simulink model "ES008A_PwrSply"  (R2013b)
settings: Solver=FixedStepDiscrete  SolverMode=SingleTasking  StartTime=0.0  StopTime=1  FixedStep=0.002  RelTol=1e-3
values from neighbouring files (symbols this model uses):
  DiagcReg0Err = DataDict.NTC    [ES008A_PwrSply_DataDict.m]
  DiagcReg1Err = DataDict.NTC    [ES008A_PwrSply_DataDict.m]
  PWRSPLYDIAGREG0READVAL_CNT_U16 = DataDict.Constant    [ES008A_PwrSply_DataDict.m]
  PWRSPLYDIAGREG1READVAL_CNT_U16 = DataDict.Constant    [ES008A_PwrSply_DataDict.m]
  PwrSplyNtc0x07BFailStep = DataDict.Calibration    [ES008A_PwrSply_DataDict.m]
  PwrSplyNtc0x07BPassStep = DataDict.Calibration    [ES008A_PwrSply_DataDict.m]
  PwrSplyNtc0x07CFailStep = DataDict.Calibration    [ES008A_PwrSply_DataDict.m]
  PwrSplyNtc0x07CPassStep = DataDict.Calibration    [ES008A_PwrSply_DataDict.m]
  PwrSplyNtc0x07DFailStep = DataDict.Calibration    [ES008A_PwrSply_DataDict.m]
  PwrSplyNtc0x07DPassStep = DataDict.Calibration    [ES008A_PwrSply_DataDict.m]
  PWRSPLYOUTPENAWRVAL_CNT_U16 = DataDict.Constant    [ES008A_PwrSply_DataDict.m]
  PWRSPLYVRFYRESREG0READVAL_CNT_U16 = DataDict.Constant    [ES008A_PwrSply_DataDict.m]
  PWRSPLYVRFYRESREG1READVAL_CNT_U16 = DataDict.Constant    [ES008A_PwrSply_DataDict.m]
  SerlErr = DataDict.NTC    [ES008A_PwrSply_DataDict.m]
  SpiConf_SpiChannel_PwrSplyCh1 = DataDict.Constant    [ES008A_PwrSply_DataDict.m]
  SpiConf_SpiChannel_PwrSplyCh2 = DataDict.Constant    [ES008A_PwrSply_DataDict.m]
  SpiConf_SpiChannel_PwrSplyCh3 = DataDict.Constant    [ES008A_PwrSply_DataDict.m]
  SpiConf_SpiChannel_PwrSplyCh4 = DataDict.Constant    [ES008A_PwrSply_DataDict.m]
  SpiConf_SpiChannel_PwrSplyCh5 = DataDict.Constant    [ES008A_PwrSply_DataDict.m]
  SpiConf_SpiSequence_PwrSplySeq1 = DataDict.Constant    [ES008A_PwrSply_DataDict.m]
  SpiConf_SpiSequence_PwrSplySeq2 = DataDict.Constant    [ES008A_PwrSply_DataDict.m]
  SpiConf_SpiSequence_PwrSplySeq3 = DataDict.Constant    [ES008A_PwrSply_DataDict.m]
  SpiConf_SpiSequence_PwrSplySeq4 = DataDict.Constant    [ES008A_PwrSply_DataDict.m]
  SpiConf_SpiSequence_PwrSplySeq5 = DataDict.Constant    [ES008A_PwrSply_DataDict.m]
  StrtUpSelfTestReg0Err = DataDict.NTC    [ES008A_PwrSply_DataDict.m]
  StrtUpSelfTestReg1Err = DataDict.NTC    [ES008A_PwrSply_DataDict.m]
undefined symbols (not defined in the file or in its folder): sigbuilder_block, SysSt1
libraries: simulink x11
(part 2 of 4)

== system ES008A_PwrSply/PwrSply/PwrSplyPer1/SysSt = Enable/PwrSplyReadWrOrderFlg1 = 1 (Read Buffer)/CH 2 // Diag Reg 0 Error - NTCNR_0X07C (V5P, V5A, V5B, V5CAN) ==
  note: Read Buffer: Temporal Monitor State
  note: Channel 2 --> for Diag Register 0
      | Channel 3 --> for Diag Register 1
  note: Diag Register 0
  Action Port : ActionPort  ActionType=then
  Chk Error : simulink/Logic and Bit Operations/Bitwise Operator  logicop=AND  UseBitMask=on  BitMask=bin2dec('11111111')  BitMaskRealWorld=Stored Integer
  Constant2 : Constant  Value=SpiConf_SpiChannel_PwrSplyCh2
  CopyRight1 : Subsystem  Description=|  mask(Copyright Information){none=on}
      | Copyright info block.                                               
      |                                                                     
      | Place copyright information at the top of every subsystem in design.
      mask prompts: none "No parameters"
      mask help: Place copyright information at the top of every subsystem in design.
      mask Display:
      | NxtrConf = 'Nexteer Confidential';
      | 
      | sys = bdroot; %handle for the current model ("system")
      | first = get_param(sys,'Created');
      | first = first(end-3:end);  %year is last four digits
      | 
      | last = get_param(sys,'LastModifiedDate');
      | if isempty(last)
      |     last = datestr(now,'yyyy');
      | else
      |     last = last(end-3:end);
      | end
      | 
      | if strcmp(first,last)
      |     fprintf('%s -- Copyright %s Nexteer',NxtrConf,first)
      | else
      |     fprintf('%s -- %s%s- %s Nexteer',NxtrConf,char(169),first,last)
      | end
  Debounce Step : Constant  Value=PwrSplyNtc0x07CFailStep  OutDataTypeStr=uint16
  NtcNr : Constant  Value=DiagcReg0Err
  NtcSts : Constant  Value=3  OutDataTypeStr=uint8
  SetNtcSts : Subsystem  RequirementInfo={'linktype_rmi_doors' '0000cf50 (/ESG Group/FDD Module Requirements/EA4 Specific/ES008A - PwrSply)' '#ES008A_90' 'true' 'REQ: ES008A_90' '' ; 'linktype_rmi_doors' '0000cf50 (/ESG Group/FDD Module Requirements/EA4 Specific/ES008A_PwrSply)' '#ES008A_111' 'true' 'REQ: ES008A_111' '' } %GIDa_0e611bfb_5a91_4369_9638_8556bad60356
  Spi_ReadIB : Subsystem  RequirementInfo={'linktype_rmi_doors' '0000cf50 (/ESG Group/FDD Module Requirements/EA4 Specific/ES008A_PwrSply)' '#ES008A_110' 'true' 'REQ: ES008A_110' '' } %GIDa_1744bced_b149_4c04_97ae_ac37b4232d20
  wires:
  NtcSts/1 -> SetNtcSts/3(NtcSts)
  Debounce Step/1 -> SetNtcSts/4(DebStep)
  NtcNr/1 -> SetNtcSts/1(NtcNr)
  Constant2/1 -> Spi_ReadIB/1(Channel)
  Spi_ReadIB/1(Rx) -> Chk Error/1
  Chk Error/1 -> SetNtcSts/2(NtcStInfo)

== system ES008A_PwrSply/PwrSply/PwrSplyPer1/SysSt = Enable/PwrSplyReadWrOrderFlg1 = 1 (Read Buffer)/CH 3 // Diag Reg 1 Error - NTCNR_0X07B (VREG, BUCK, V3V3) ==
  note: Channel 2 --> for Diag Register 0
      | Channel 3 --> for Diag Register 1
  note: Read Buffer: Temporal Monitor State
  note: Diag Register 1
  Action Port : ActionPort  ActionType=then
  Chk Error : simulink/Logic and Bit Operations/Bitwise Operator  logicop=AND  UseBitMask=on  BitMask=bin2dec('00111111')  BitMaskRealWorld=Stored Integer
  Constant2 : Constant  Value=SpiConf_SpiChannel_PwrSplyCh3
  CopyRight1 : Subsystem  Description=|  mask(Copyright Information){none=on}
      | Copyright info block.                                               
      |                                                                     
      | Place copyright information at the top of every subsystem in design.
      mask prompts: none "No parameters"
      mask help: Place copyright information at the top of every subsystem in design.
      mask Display:
      | NxtrConf = 'Nexteer Confidential';
      | 
      | sys = bdroot; %handle for the current model ("system")
      | first = get_param(sys,'Created');
      | first = first(end-3:end);  %year is last four digits
      | 
      | last = get_param(sys,'LastModifiedDate');
      | if isempty(last)
      |     last = datestr(now,'yyyy');
      | else
      |     last = last(end-3:end);
      | end
      | 
      | if strcmp(first,last)
      |     fprintf('%s -- Copyright %s Nexteer',NxtrConf,first)
      | else
      |     fprintf('%s -- %s%s- %s Nexteer',NxtrConf,char(169),first,last)
      | end
  Debounce Step : Constant  Value=PwrSplyNtc0x07BFailStep  OutDataTypeStr=uint16
  NtcNr : Constant  Value=DiagcReg1Err
  NtcSts : Constant  Value=3  OutDataTypeStr=uint8
  SetNtcSts : Subsystem  RequirementInfo={'linktype_rmi_doors' '0000cf50 (/ESG Group/FDD Module Requirements/EA4 Specific/ES008A - PwrSply)' '#ES008A_22' 'true' 'REQ: ES008A_22' '' ; 'linktype_rmi_doors' '0000cf50 (/ESG Group/FDD Module Requirements/EA4 Specific/ES008A_PwrSply)' '#ES008A_111' 'true' 'REQ: ES008A_111' '' } %GIDa_0332d9c1_390b_4a00_b6d5_767a4bc1c83a
  Spi_ReadIB : Subsystem  RequirementInfo={'linktype_rmi_doors' '0000cf50 (/ESG Group/FDD Module Requirements/EA4 Specific/ES008A_PwrSply)' '#ES008A_110' 'true' 'REQ: ES008A_110' '' } %GIDa_30f8a1e3_071e_4be7_af63_a65be91c4651
  wires:
  Chk Error/1 -> SetNtcSts/2(NtcStInfo)
  Spi_ReadIB/1(Rx) -> Chk Error/1
  Constant2/1 -> Spi_ReadIB/1(Channel)
  NtcNr/1 -> SetNtcSts/1(NtcNr)
  Debounce Step/1 -> SetNtcSts/4(DebStep)
  NtcSts/1 -> SetNtcSts/3(NtcSts)

== system ES008A_PwrSply/PwrSply/PwrSplyPer1/SysSt = Enable/PwrSplyReadWrOrderFlg1 = 1 (Read Buffer)/CopyRight1 ==

== system ES008A_PwrSply/PwrSply/PwrSplyPer1/SysSt = Enable/PwrSplyReadWrOrderFlg1 = 1 (Read Buffer)/No  Error - Diag Reg 0 ==
  Action Port : ActionPort  ActionType=else
  CopyRight1 : Subsystem  Description=|  mask(Copyright Information){none=on}
      | Copyright info block.                                               
      |                                                                     
      | Place copyright information at the top of every subsystem in design.
      mask prompts: none "No parameters"
      mask help: Place copyright information at the top of every subsystem in design.
      mask Display:
      | NxtrConf = 'Nexteer Confidential';
      | 
      | sys = bdroot; %handle for the current model ("system")
      | first = get_param(sys,'Created');
      | first = first(end-3:end);  %year is last four digits
      | 
      | last = get_param(sys,'LastModifiedDate');
      | if isempty(last)
      |     last = datestr(now,'yyyy');
      | else
      |     last = last(end-3:end);
      | end
      | 
      | if strcmp(first,last)
      |     fprintf('%s -- Copyright %s Nexteer',NxtrConf,first)
      | else
      |     fprintf('%s -- %s%s- %s Nexteer',NxtrConf,char(169),first,last)
      | end
  Debounce Step : Constant  Value=PwrSplyNtc0x07CPassStep  OutDataTypeStr=uint16
  NtcNr : Constant  Value=DiagcReg0Err
  NtcSts : Constant  Value=2  OutDataTypeStr=uint8
  NtcStsInfo : Constant  Value=0  OutDataTypeStr=uint8
  SetNtcSts : Subsystem
  wires:
  NtcSts/1 -> SetNtcSts/3(NtcSts)
  Debounce Step/1 -> SetNtcSts/4(DebStep)
  NtcNr/1 -> SetNtcSts/1(NtcNr)
  NtcStsInfo/1 -> SetNtcSts/2(NtcStInfo)

== system ES008A_PwrSply/PwrSply/PwrSplyPer1/SysSt = Enable/PwrSplyReadWrOrderFlg1 = 1 (Read Buffer)/No  Error - Diag Reg 1 ==
  Action Port : ActionPort  ActionType=else
  CopyRight1 : Subsystem  Description=|  mask(Copyright Information){none=on}
      | Copyright info block.                                               
      |                                                                     
      | Place copyright information at the top of every subsystem in design.
      mask prompts: none "No parameters"
      mask help: Place copyright information at the top of every subsystem in design.
      mask Display:
      | NxtrConf = 'Nexteer Confidential';
      | 
      | sys = bdroot; %handle for the current model ("system")
      | first = get_param(sys,'Created');
      | first = first(end-3:end);  %year is last four digits
      | 
      | last = get_param(sys,'LastModifiedDate');
      | if isempty(last)
      |     last = datestr(now,'yyyy');
      | else
      |     last = last(end-3:end);
      | end
      | 
      | if strcmp(first,last)
      |     fprintf('%s -- Copyright %s Nexteer',NxtrConf,first)
      | else
      |     fprintf('%s -- %s%s- %s Nexteer',NxtrConf,char(169),first,last)
      | end
  Debounce Step : Constant  Value=PwrSplyNtc0x07BPassStep  OutDataTypeStr=uint16
  NtcNr : Constant  Value=DiagcReg1Err
  NtcSts : Constant  Value=2  OutDataTypeStr=uint8
  NtcStsInfo : Constant  Value=0  OutDataTypeStr=uint8
  SetNtcSts : Subsystem
  wires:
  NtcStsInfo/1 -> SetNtcSts/2(NtcStInfo)
  NtcNr/1 -> SetNtcSts/1(NtcNr)
  Debounce Step/1 -> SetNtcSts/4(DebStep)
  NtcSts/1 -> SetNtcSts/3(NtcSts)

== system ES008A_PwrSply/PwrSply/PwrSplyPer1/SysSt = Enable/PwrSplyReadWrOrderFlg1 = 1 (Read Buffer)/No Serial Error ==
  Action Port : ActionPort  ActionType=else
  CopyRight1 : Subsystem  Description=|  mask(Copyright Information){none=on}
      | Copyright info block.                                               
      |                                                                     
      | Place copyright information at the top of every subsystem in design.
      mask prompts: none "No parameters"
      mask help: Place copyright information at the top of every subsystem in design.
      mask Display:
      | NxtrConf = 'Nexteer Confidential';
      | 
      | sys = bdroot; %handle for the current model ("system")
      | first = get_param(sys,'Created');
      | first = first(end-3:end);  %year is last four digits
      | 
      | last = get_param(sys,'LastModifiedDate');
      | if isempty(last)
      |     last = datestr(now,'yyyy');
      | else
      |     last = last(end-3:end);
      | end
      | 
      | if strcmp(first,last)
      |     fprintf('%s -- Copyright %s Nexteer',NxtrConf,first)
      | else
      |     fprintf('%s -- %s%s- %s Nexteer',NxtrConf,char(169),first,last)
      | end
  Debounce Step : Constant  Value=PwrSplyNtc0x07DPassStep  OutDataTypeStr=uint16
  NtcNr : Constant  Value=SerlErr
  NtcSts : Constant  Value=2  OutDataTypeStr=uint8
  NtcStsInfo : Constant  Value=0  OutDataTypeStr=uint8
  SetNtcSts : Subsystem
  wires:
  NtcSts/1 -> SetNtcSts/3(NtcSts)
  Debounce Step/1 -> SetNtcSts/4(DebStep)
  NtcNr/1 -> SetNtcSts/1(NtcNr)
  NtcStsInfo/1 -> SetNtcSts/2(NtcStInfo)

== system ES008A_PwrSply/PwrSply/PwrSplyPer1/SysSt = Enable/PwrSplyReadWrOrderFlg1 = 1 (Read Buffer)/Serial Error - NTCNR_0X07D ==
  Action Port : ActionPort  ActionType=then
  CopyRight1 : Subsystem  Description=|  mask(Copyright Information){none=on}
      | Copyright info block.                                               
      |                                                                     
      | Place copyright information at the top of every subsystem in design.
      mask prompts: none "No parameters"
      mask help: Place copyright information at the top of every subsystem in design.
      mask Display:
      | NxtrConf = 'Nexteer Confidential';
      | 
      | sys = bdroot; %handle for the current model ("system")
      | first = get_param(sys,'Created');
      | first = first(end-3:end);  %year is last four digits
      | 
      | last = get_param(sys,'LastModifiedDate');
      | if isempty(last)
      |     last = datestr(now,'yyyy');
      | else
      |     last = last(end-3:end);
      | end
      | 
      | if strcmp(first,last)
      |     fprintf('%s -- Copyright %s Nexteer',NxtrConf,first)
      | else
      |     fprintf('%s -- %s%s- %s Nexteer',NxtrConf,char(169),first,last)
      | end
  Debounce Step : Constant  Value=PwrSplyNtc0x07DFailStep  OutDataTypeStr=uint16
  NtcNr : Constant  Value=SerlErr
  NtcSts : Constant  Value=3  OutDataTypeStr=uint8
  NtcSts1 : Constant  OutDataTypeStr=uint8
  SetNtcSts : Subsystem  RequirementInfo={'linktype_rmi_doors' '0000cf50 (/ESG Group/FDD Module Requirements/EA4 Specific/ES008A - PwrSply)' '#ES008A_96' 'true' 'REQ: ES008A_96' '' } %GIDa_f352822b_41ef_4404_b4d0_7ec6dffd63c0
  wires:
  NtcSts/1 -> SetNtcSts/3(NtcSts)
  Debounce Step/1 -> SetNtcSts/4(DebStep)
  NtcNr/1 -> SetNtcSts/1(NtcNr)
  NtcSts1/1 -> SetNtcSts/2(NtcStInfo)

== system ES008A_PwrSply/PwrSply/PwrSplyPer1/SysSt = Enable/PwrSplyReadWrOrderFlg1 = 1 (Read Buffer)/Spi_ReadIB ==
  note: 001011111111110
  note: Read Buffer - Simulation Purpose Only
  Channel : Inport
  Constant3 : Constant  Value=44  OutDataTypeStr=uint16
  CopyRight1 : Subsystem  Description=|  mask(Copyright Information){none=on}
      | Copyright info block.                                               
      |                                                                     
      | Place copyright information at the top of every subsystem in design.
      mask prompts: none "No parameters"
      mask help: Place copyright information at the top of every subsystem in design.
      mask Display:
      | NxtrConf = 'Nexteer Confidential';
      | 
      | sys = bdroot; %handle for the current model ("system")
      | first = get_param(sys,'Created');
      | first = first(end-3:end);  %year is last four digits
      | 
      | last = get_param(sys,'LastModifiedDate');
      | if isempty(last)
      |     last = datestr(now,'yyyy');
      | else
      |     last = last(end-3:end);
      | end
      | 
      | if strcmp(first,last)
      |     fprintf('%s -- Copyright %s Nexteer',NxtrConf,first)
      | else
      |     fprintf('%s -- %s%s- %s Nexteer',NxtrConf,char(169),first,last)
      | end
  Terminator : Terminator
  Rx : Outport
  wires:
  Constant3/1 -> Rx/1
  Channel/1 -> Terminator/1

== system ES008A_PwrSply/PwrSply/PwrSplyPer1/SysSt = Warm Init OR Enable/PwrSplyReadWrOrderFlg2 = 0 (Write Cmd to get Diag Status) /CopyRight1 ==

== system ES008A_PwrSply/PwrSply/PwrSplyPer1/SysSt = Warm Init OR Enable/PwrSplyReadWrOrderFlg2 = 0 (Write Cmd to get Diag Status) /Read Message 1 ==
  note: Read Cmd: Diag Reg 0: 01010 0 0 00000000 P
  note: Channel 4 --> for Verify_Result_0 Register
      | Channel 5 --> for Verify_Result_1 Register
  note: 10240
  Call_Spi_AsyncTransmit : Subsystem
  Constant2 : Constant  Value=SpiConf_SpiSequence_PwrSplySeq4
  Constant3 : Constant  Value=SpiConf_SpiChannel_PwrSplyCh4
  Constant5 : Constant  Value=PWRSPLYVRFYRESREG0READVAL_CNT_U16
  CopyRight1 : Subsystem  Description=|  mask(Copyright Information){none=on}
      | Copyright info block.                                               
      |                                                                     
      | Place copyright information at the top of every subsystem in design.
      mask prompts: none "No parameters"
      mask help: Place copyright information at the top of every subsystem in design.
      mask Display:
      | NxtrConf = 'Nexteer Confidential';
      | 
      | sys = bdroot; %handle for the current model ("system")
      | first = get_param(sys,'Created');
      | first = first(end-3:end);  %year is last four digits
      | 
      | last = get_param(sys,'LastModifiedDate');
      | if isempty(last)
      |     last = datestr(now,'yyyy');
      | else
      |     last = last(end-3:end);
      | end
      | 
      | if strcmp(first,last)
      |     fprintf('%s -- Copyright %s Nexteer',NxtrConf,first)
      | else
      |     fprintf('%s -- %s%s- %s Nexteer',NxtrConf,char(169),first,last)
      | end
  Spi_WriteIB : Subsystem
  wires:
  Constant3/1 -> Spi_WriteIB/1(Channel)
  Constant5/1 -> Spi_WriteIB/2(DataBufferPtr)
  Constant2/1 -> Call_Spi_AsyncTransmit/1(Sequence)

== system ES008A_PwrSply/PwrSply/PwrSplyPer1/SysSt = Warm Init OR Enable/PwrSplyReadWrOrderFlg2 = 0 (Write Cmd to get Diag Status) /Read Message 2 ==
  note: Channel 4 --> for Verify_Result_0 Register
      | Channel 5 --> for Verify_Result_1 Register
  note: Read Cmd: Diag Reg 0: 01011 0 0 00000000 P
  note: 11264
  Call_Spi_AsyncTransmit : Subsystem
  Constant10 : Constant  Value=PWRSPLYVRFYRESREG1READVAL_CNT_U16
  Constant8 : Constant  Value=SpiConf_SpiSequence_PwrSplySeq5
  Constant9 : Constant  Value=SpiConf_SpiChannel_PwrSplyCh5
  CopyRight1 : Subsystem  Description=|  mask(Copyright Information){none=on}
      | Copyright info block.                                               
      |                                                                     
      | Place copyright information at the top of every subsystem in design.
      mask prompts: none "No parameters"
      mask help: Place copyright information at the top of every subsystem in design.
      mask Display:
      | NxtrConf = 'Nexteer Confidential';
      | 
      | sys = bdroot; %handle for the current model ("system")
      | first = get_param(sys,'Created');
      | first = first(end-3:end);  %year is last four digits
      | 
      | last = get_param(sys,'LastModifiedDate');
      | if isempty(last)
      |     last = datestr(now,'yyyy');
      | else
      |     last = last(end-3:end);
      | end
      | 
      | if strcmp(first,last)
      |     fprintf('%s -- Copyright %s Nexteer',NxtrConf,first)
      | else
      |     fprintf('%s -- %s%s- %s Nexteer',NxtrConf,char(169),first,last)
      | end
  Spi_WriteIB : Subsystem
  wires:
  Constant9/1 -> Spi_WriteIB/1(Channel)
  Constant10/1 -> Spi_WriteIB/2(DataBufferPtr)
  Constant8/1 -> Call_Spi_AsyncTransmit/1(Sequence)

== system ES008A_PwrSply/PwrSply/PwrSplyPer1/SysSt = Warm Init OR Enable/PwrSplyReadWrOrderFlg2 = 1 (Read Buffer)/Channel 4 ==
  note: Read Buffer: Temporal Monitor State
  "CH 4 / Verify Result Reg 0 - NTCNR_0X07E (V5A, V5CAN, 3V3, BUCK)" : Subsystem  RequirementInfo={} %GIDa_cbb4265b_4cf8_442f_858d_d36cb4b86b78
  Ch 4 Mask : simulink/Logic and Bit Operations/Bitwise Operator  logicop=AND  UseBitMask=on  BitMask=bin2dec('11111111')  BitMaskRealWorld=Stored Integer
  Constant2 : Constant  Value=SpiConf_SpiChannel_PwrSplyCh4
  CopyRight1 : Subsystem  Description=|  mask(Copyright Information){none=on}
      | Copyright info block.                                               
      |                                                                     
      | Place copyright information at the top of every subsystem in design.
      mask prompts: none "No parameters"
      mask help: Place copyright information at the top of every subsystem in design.
      mask Display:
      | NxtrConf = 'Nexteer Confidential';
      | 
      | sys = bdroot; %handle for the current model ("system")
      | first = get_param(sys,'Created');
      | first = first(end-3:end);  %year is last four digits
      | 
      | last = get_param(sys,'LastModifiedDate');
      | if isempty(last)
      |     last = datestr(now,'yyyy');
      | else
      |     last = last(end-3:end);
      | end
      | 
      | if strcmp(first,last)
      |     fprintf('%s -- Copyright %s Nexteer',NxtrConf,first)
      | else
      |     fprintf('%s -- %s%s- %s Nexteer',NxtrConf,char(169),first,last)
      | end
  Data Type Conversion : DataTypeConversion  OutDataTypeStr=uint8
  If1 : If  IfExpression=u1 ~= 255
  No Startup Test Error 0 : Subsystem  RequirementInfo={} %GIDa_3b3e5102_6261_4158_b35c_23f9e2a3cb68
  Spi_ReadIB : Subsystem
  wires:
  If1/2 -> No Startup Test Error 0/Action
  If1/1 -> "CH 4 / Verify Result Reg 0 - NTCNR_0X07E (V5A, V5CAN, 3V3, BUCK)"/Action
  Constant2/1 -> Spi_ReadIB/1(Channel)
  Spi_ReadIB/1(Rx) -> Ch 4 Mask/1
  Ch 4 Mask/1 -> Data Type Conversion/1, If1/1
  Data Type Conversion/1 -> "CH 4 / Verify Result Reg 0 - NTCNR_0X07E (V5A, V5CAN, 3V3, BUCK)"/1(NtcStsInfo)

== system ES008A_PwrSply/PwrSply/PwrSplyPer1/SysSt = Warm Init OR Enable/PwrSplyReadWrOrderFlg2 = 1 (Read Buffer)/Channel 5 ==
  note: Read Buffer: Temporal Monitor State
  "CH 5 / Verify Result Reg 1 - NTCNR_0X07F (VREG, V5P, V5B)" : Subsystem  RequirementInfo={} %GIDa_ed8a5c25_78d9_457b_8dd9_ed5061905495
  Ch 5 Mask : simulink/Logic and Bit Operations/Bitwise Operator  logicop=AND  UseBitMask=on  BitMask=bin2dec('00111111')  BitMaskRealWorld=Stored Integer
  Constant3 : Constant  Value=SpiConf_SpiChannel_PwrSplyCh5
  CopyRight1 : Subsystem  Description=|  mask(Copyright Information){none=on}
      | Copyright info block.                                               
      |                                                                     
      | Place copyright information at the top of every subsystem in design.
      mask prompts: none "No parameters"
      mask help: Place copyright information at the top of every subsystem in design.
      mask Display:
      | NxtrConf = 'Nexteer Confidential';
      | 
      | sys = bdroot; %handle for the current model ("system")
      | first = get_param(sys,'Created');
      | first = first(end-3:end);  %year is last four digits
      | 
      | last = get_param(sys,'LastModifiedDate');
      | if isempty(last)
      |     last = datestr(now,'yyyy');
      | else
      |     last = last(end-3:end);
      | end
      | 
      | if strcmp(first,last)
      |     fprintf('%s -- Copyright %s Nexteer',NxtrConf,first)
      | else
      |     fprintf('%s -- %s%s- %s Nexteer',NxtrConf,char(169),first,last)
      | end
  Data Type Conversion : DataTypeConversion  OutDataTypeStr=uint8
  If2 : If  IfExpression=u1 ~= 63
  No Startup Test Error 1 : Subsystem  RequirementInfo={} %GIDa_2f0cd04e_2890_4518_8b5f_f24d207f9195
  Spi_ReadIB : Subsystem
  wires:
  If2/2 -> No Startup Test Error 1/Action
  If2/1 -> "CH 5 / Verify Result Reg 1 - NTCNR_0X07F (VREG, V5P, V5B)"/Action
  Ch 5 Mask/1 -> Data Type Conversion/1, If2/1
  Constant3/1 -> Spi_ReadIB/1(Channel)
  Spi_ReadIB/1(Rx) -> Ch 5 Mask/1
  Data Type Conversion/1 -> "CH 5 / Verify Result Reg 1 - NTCNR_0X07F (VREG, V5P, V5B)"/1(NtcStsInfo)

== system ES008A_PwrSply/PwrSply/PwrSplyPer1/SysSt = Warm Init OR Enable/PwrSplyReadWrOrderFlg2 = 1 (Read Buffer)/CopyRight1 ==

== system ES008A_PwrSply/PwrSply/PwrSplyPer1/SysSt = Enable/PwrSplyReadWrOrderFlg1 = 0 (Write Cmd to get Diag Status) /Read Message 1/Call_Spi_AsyncTransmit ==
  Sequence : Inport
  CopyRight1 : Subsystem  Description=|  mask(Copyright Information){none=on}
      | Copyright info block.                                               
      |                                                                     
      | Place copyright information at the top of every subsystem in design.
      mask prompts: none "No parameters"
      mask help: Place copyright information at the top of every subsystem in design.
      mask Display:
      | NxtrConf = 'Nexteer Confidential';
      | 
      | sys = bdroot; %handle for the current model ("system")
      | first = get_param(sys,'Created');
      | first = first(end-3:end);  %year is last four digits
      | 
      | last = get_param(sys,'LastModifiedDate');
      | if isempty(last)
      |     last = datestr(now,'yyyy');
      | else
      |     last = last(end-3:end);
      | end
      | 
      | if strcmp(first,last)
      |     fprintf('%s -- Copyright %s Nexteer',NxtrConf,first)
      | else
      |     fprintf('%s -- %s%s- %s Nexteer',NxtrConf,char(169),first,last)
      | end
  Terminator : Terminator
  wires:
  Sequence/1 -> Terminator/1

== system ES008A_PwrSply/PwrSply/PwrSplyPer1/SysSt = Enable/PwrSplyReadWrOrderFlg1 = 0 (Write Cmd to get Diag Status) /Read Message 1/CopyRight1 ==

== system ES008A_PwrSply/PwrSply/PwrSplyPer1/SysSt = Enable/PwrSplyReadWrOrderFlg1 = 0 (Write Cmd to get Diag Status) /Read Message 1/Spi_WriteIB ==
  Channel : Inport
  DataBufferPtr : Inport  Port=2
  CopyRight1 : Subsystem  Description=|  mask(Copyright Information){none=on}
      | Copyright info block.                                               
      |                                                                     
      | Place copyright information at the top of every subsystem in design.
      mask prompts: none "No parameters"
      mask help: Place copyright information at the top of every subsystem in design.
      mask Display:
      | NxtrConf = 'Nexteer Confidential';
      | 
      | sys = bdroot; %handle for the current model ("system")
      | first = get_param(sys,'Created');
      | first = first(end-3:end);  %year is last four digits
      | 
      | last = get_param(sys,'LastModifiedDate');
      | if isempty(last)
      |     last = datestr(now,'yyyy');
      | else
      |     last = last(end-3:end);
      | end
      | 
      | if strcmp(first,last)
      |     fprintf('%s -- Copyright %s Nexteer',NxtrConf,first)
      | else
      |     fprintf('%s -- %s%s- %s Nexteer',NxtrConf,char(169),first,last)
      | end
  Terminator : Terminator
  Terminator1 : Terminator
  wires:
  Channel/1 -> Terminator/1
  DataBufferPtr/1 -> Terminator1/1

== system ES008A_PwrSply/PwrSply/PwrSplyPer1/SysSt = Enable/PwrSplyReadWrOrderFlg1 = 0 (Write Cmd to get Diag Status) /Read Message 2/Call_Spi_AsyncTransmit ==
  Sequence : Inport
  CopyRight1 : Subsystem  Description=|  mask(Copyright Information){none=on}
      | Copyright info block.                                               
      |                                                                     
      | Place copyright information at the top of every subsystem in design.
      mask prompts: none "No parameters"
      mask help: Place copyright information at the top of every subsystem in design.
      mask Display:
      | NxtrConf = 'Nexteer Confidential';
      | 
      | sys = bdroot; %handle for the current model ("system")
      | first = get_param(sys,'Created');
      | first = first(end-3:end);  %year is last four digits
      | 
      | last = get_param(sys,'LastModifiedDate');
      | if isempty(last)
      |     last = datestr(now,'yyyy');
      | else
      |     last = last(end-3:end);
      | end
      | 
      | if strcmp(first,last)
      |     fprintf('%s -- Copyright %s Nexteer',NxtrConf,first)
      | else
      |     fprintf('%s -- %s%s- %s Nexteer',NxtrConf,char(169),first,last)
      | end
  Terminator : Terminator
  wires:
  Sequence/1 -> Terminator/1

== system ES008A_PwrSply/PwrSply/PwrSplyPer1/SysSt = Enable/PwrSplyReadWrOrderFlg1 = 0 (Write Cmd to get Diag Status) /Read Message 2/CopyRight1 ==

== system ES008A_PwrSply/PwrSply/PwrSplyPer1/SysSt = Enable/PwrSplyReadWrOrderFlg1 = 0 (Write Cmd to get Diag Status) /Read Message 2/Spi_WriteIB ==
  Channel : Inport
  DataBufferPtr : Inport  Port=2
  CopyRight1 : Subsystem  Description=|  mask(Copyright Information){none=on}
      | Copyright info block.                                               
      |                                                                     
      | Place copyright information at the top of every subsystem in design.
      mask prompts: none "No parameters"
      mask help: Place copyright information at the top of every subsystem in design.
      mask Display:
      | NxtrConf = 'Nexteer Confidential';
      | 
      | sys = bdroot; %handle for the current model ("system")
      | first = get_param(sys,'Created');
      | first = first(end-3:end);  %year is last four digits
      | 
      | last = get_param(sys,'LastModifiedDate');
      | if isempty(last)
      |     last = datestr(now,'yyyy');
      | else
      |     last = last(end-3:end);
      | end
      | 
      | if strcmp(first,last)
      |     fprintf('%s -- Copyright %s Nexteer',NxtrConf,first)
      | else
      |     fprintf('%s -- %s%s- %s Nexteer',NxtrConf,char(169),first,last)
      | end
  Terminator : Terminator
  Terminator1 : Terminator
  wires:
  DataBufferPtr/1 -> Terminator1/1
  Channel/1 -> Terminator/1

== system ES008A_PwrSply/PwrSply/PwrSplyPer1/SysSt = Enable/PwrSplyReadWrOrderFlg1 = 0 (Write Cmd to get Diag Status) /Write Message 1/Call_Spi_AsyncTransmit ==
  Sequence : Inport
  CopyRight1 : Subsystem  Description=|  mask(Copyright Information){none=on}
      | Copyright info block.                                               
      |                                                                     
      | Place copyright information at the top of every subsystem in design.
      mask prompts: none "No parameters"
      mask help: Place copyright information at the top of every subsystem in design.
      mask Display:
      | NxtrConf = 'Nexteer Confidential';
      | 
      | sys = bdroot; %handle for the current model ("system")
      | first = get_param(sys,'Created');
      | first = first(end-3:end);  %year is last four digits
      | 
      | last = get_param(sys,'LastModifiedDate');
      | if isempty(last)
      |     last = datestr(now,'yyyy');
      | else
      |     last = last(end-3:end);
      | end
      | 
      | if strcmp(first,last)
      |     fprintf('%s -- Copyright %s Nexteer',NxtrConf,first)
      | else
      |     fprintf('%s -- %s%s- %s Nexteer',NxtrConf,char(169),first,last)
      | end
  Terminator : Terminator
  wires:
  Sequence/1 -> Terminator/1

== system ES008A_PwrSply/PwrSply/PwrSplyPer1/SysSt = Enable/PwrSplyReadWrOrderFlg1 = 0 (Write Cmd to get Diag Status) /Write Message 1/CopyRight1 ==

== system ES008A_PwrSply/PwrSply/PwrSplyPer1/SysSt = Enable/PwrSplyReadWrOrderFlg1 = 0 (Write Cmd to get Diag Status) /Write Message 1/Spi_WriteIB ==
  Channel : Inport
  DataBufferPtr : Inport  Port=2
  CopyRight1 : Subsystem  Description=|  mask(Copyright Information){none=on}
      | Copyright info block.                                               
      |                                                                     
      | Place copyright information at the top of every subsystem in design.
      mask prompts: none "No parameters"
      mask help: Place copyright information at the top of every subsystem in design.
      mask Display:
      | NxtrConf = 'Nexteer Confidential';
      | 
      | sys = bdroot; %handle for the current model ("system")
      | first = get_param(sys,'Created');
      | first = first(end-3:end);  %year is last four digits
      | 
      | last = get_param(sys,'LastModifiedDate');
      | if isempty(last)
      |     last = datestr(now,'yyyy');
      | else
      |     last = last(end-3:end);
      | end
      | 
      | if strcmp(first,last)
      |     fprintf('%s -- Copyright %s Nexteer',NxtrConf,first)
      | else
      |     fprintf('%s -- %s%s- %s Nexteer',NxtrConf,char(169),first,last)
      | end
  Terminator : Terminator
  Terminator1 : Terminator
  wires:
  Channel/1 -> Terminator/1
  DataBufferPtr/1 -> Terminator1/1

== system ES008A_PwrSply/PwrSply/PwrSplyPer1/SysSt = Enable/PwrSplyReadWrOrderFlg1 = 1 (Read Buffer)/CH 2 // Diag Reg 0 Error - NTCNR_0X07C (V5P, V5A, V5B, V5CAN)/CopyRight1 ==

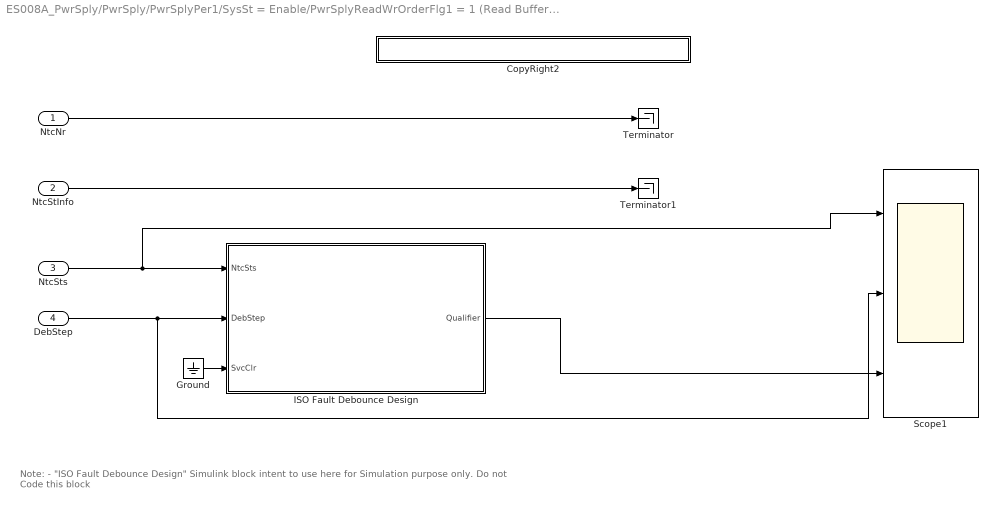
== system ES008A_PwrSply/PwrSply/PwrSplyPer1/SysSt = Enable/PwrSplyReadWrOrderFlg1 = 1 (Read Buffer)/CH 2 // Diag Reg 0 Error - NTCNR_0X07C (V5P, V5A, V5B, V5CAN)/SetNtcSts ==
  note: Note:
      |
      | - "ISO Fault Debounce Design" Simulink block intent to use here for Simulation purpose only. Do not Code this block
  NtcNr : Inport
  NtcStInfo : Inport  Port=2
  NtcSts : Inport  Port=3  OutDataTypeStr=uint8
  DebStep : Inport  Port=4  OutDataTypeStr=uint16
  CopyRight2 : Subsystem  Description=|  mask(Copyright Information){none=on}
      | Copyright info block.                                               
      |                                                                     
      | Place copyright information at the top of every subsystem in design.
      mask prompts: none "No parameters"
      mask help: Place copyright information at the top of every subsystem in design.
      mask Display:
      | NxtrConf = 'Nexteer Confidential';
      | 
      | sys = bdroot; %handle for the current model ("system")
      | first = get_param(sys,'Created');
      | first = first(end-3:end);  %year is last four digits
      | 
      | last = get_param(sys,'LastModifiedDate');
      | if isempty(last)
      |     last = datestr(now,'yyyy');
      | else
      |     last = last(end-3:end);
      | end
      | 
      | if strcmp(first,last)
      |     fprintf('%s -- Copyright %s Nexteer',NxtrConf,first)
      | else
      |     fprintf('%s -- %s%s- %s Nexteer',NxtrConf,char(169),first,last)
      | end
  Ground : Ground
  ISO Fault Debounce Design : Stateflow chart  TreatAsAtomicUnit=on
      settings: AttributesFormatString=|
      | Simulation Purpose Only.
      | Do Not Code this block
      | Diagnostic Manager Owns this requirement
  Scope1 : Scope  NumInputPorts=3
      settings: YMin=-5~-5~-5  YMax=5~5~5  SaveName=ScopeData5
  Terminator : Terminator
  Terminator1 : Terminator
  wires:
  Ground/1 -> ISO Fault Debounce Design/3(SvcClr)
  ISO Fault Debounce Design/1(Qualifier) -> Scope1/3
  DebStep/1 -> Scope1/2, ISO Fault Debounce Design/2(DebStep)
  NtcSts/1 -> Scope1/1, ISO Fault Debounce Design/1(NtcSts)
  NtcNr/1 -> Terminator/1
  NtcStInfo/1 -> Terminator1/1

== system ES008A_PwrSply/PwrSply/PwrSplyPer1/SysSt = Enable/PwrSplyReadWrOrderFlg1 = 1 (Read Buffer)/CH 2 // Diag Reg 0 Error - NTCNR_0X07C (V5P, V5A, V5B, V5CAN)/Spi_ReadIB ==
  note: Read Buffer - Simulation Purpose Only
  note: 00000000
  Channel : Inport
  Constant3 : Constant  Value=44  OutDataTypeStr=uint16
  CopyRight1 : Subsystem  Description=|  mask(Copyright Information){none=on}
      | Copyright info block.                                               
      |                                                                     
      | Place copyright information at the top of every subsystem in design.
      mask prompts: none "No parameters"
      mask help: Place copyright information at the top of every subsystem in design.
      mask Display:
      | NxtrConf = 'Nexteer Confidential';
      | 
      | sys = bdroot; %handle for the current model ("system")
      | first = get_param(sys,'Created');
      | first = first(end-3:end);  %year is last four digits
      | 
      | last = get_param(sys,'LastModifiedDate');
      | if isempty(last)
      |     last = datestr(now,'yyyy');
      | else
      |     last = last(end-3:end);
      | end
      | 
      | if strcmp(first,last)
      |     fprintf('%s -- Copyright %s Nexteer',NxtrConf,first)
      | else
      |     fprintf('%s -- %s%s- %s Nexteer',NxtrConf,char(169),first,last)
      | end
  Terminator : Terminator
  Rx : Outport
  wires:
  Channel/1 -> Terminator/1
  Constant3/1 -> Rx/1

== system ES008A_PwrSply/PwrSply/PwrSplyPer1/SysSt = Enable/PwrSplyReadWrOrderFlg1 = 1 (Read Buffer)/CH 3 // Diag Reg 1 Error - NTCNR_0X07B (VREG, BUCK, V3V3)/CopyRight1 ==

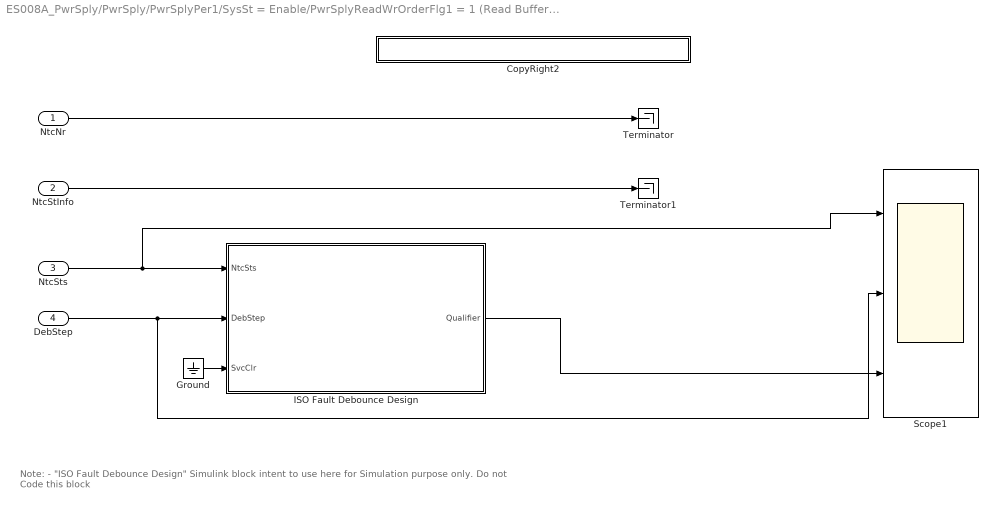
== system ES008A_PwrSply/PwrSply/PwrSplyPer1/SysSt = Enable/PwrSplyReadWrOrderFlg1 = 1 (Read Buffer)/CH 3 // Diag Reg 1 Error - NTCNR_0X07B (VREG, BUCK, V3V3)/SetNtcSts ==
  note: Note:
      |
      | - "ISO Fault Debounce Design" Simulink block intent to use here for Simulation purpose only. Do not Code this block
  NtcNr : Inport
  NtcStInfo : Inport  Port=2
  NtcSts : Inport  Port=3  OutDataTypeStr=uint8
  DebStep : Inport  Port=4  OutDataTypeStr=uint16
  CopyRight2 : Subsystem  Description=|  mask(Copyright Information){none=on}
      | Copyright info block.                                               
      |                                                                     
      | Place copyright information at the top of every subsystem in design.
      mask prompts: none "No parameters"
      mask help: Place copyright information at the top of every subsystem in design.
      mask Display:
      | NxtrConf = 'Nexteer Confidential';
      | 
      | sys = bdroot; %handle for the current model ("system")
      | first = get_param(sys,'Created');
      | first = first(end-3:end);  %year is last four digits
      | 
      | last = get_param(sys,'LastModifiedDate');
      | if isempty(last)
      |     last = datestr(now,'yyyy');
      | else
      |     last = last(end-3:end);
      | end
      | 
      | if strcmp(first,last)
      |     fprintf('%s -- Copyright %s Nexteer',NxtrConf,first)
      | else
      |     fprintf('%s -- %s%s- %s Nexteer',NxtrConf,char(169),first,last)
      | end
  Ground : Ground
  ISO Fault Debounce Design : Stateflow chart  TreatAsAtomicUnit=on
      settings: AttributesFormatString=|
      | Simulation Purpose Only.
      | Do Not Code this block
      | Diagnostic Manager Owns this requirement
  Scope1 : Scope  NumInputPorts=3
      settings: YMin=-5~-5~-5  YMax=5~5~5  SaveName=ScopeData5
  Terminator : Terminator
  Terminator1 : Terminator
  wires:
  NtcStInfo/1 -> Terminator1/1
  NtcNr/1 -> Terminator/1
  NtcSts/1 -> ISO Fault Debounce Design/1(NtcSts), Scope1/1
  DebStep/1 -> ISO Fault Debounce Design/2(DebStep), Scope1/2
  ISO Fault Debounce Design/1(Qualifier) -> Scope1/3
  Ground/1 -> ISO Fault Debounce Design/3(SvcClr)

== system ES008A_PwrSply/PwrSply/PwrSplyPer1/SysSt = Enable/PwrSplyReadWrOrderFlg1 = 1 (Read Buffer)/CH 3 // Diag Reg 1 Error - NTCNR_0X07B (VREG, BUCK, V3V3)/Spi_ReadIB ==
  note: 00000000
  note: Read Buffer - Simulation Purpose Only
  Channel : Inport
  Constant3 : Constant  Value=44  OutDataTypeStr=uint16
  CopyRight1 : Subsystem  Description=|  mask(Copyright Information){none=on}
      | Copyright info block.                                               
      |                                                                     
      | Place copyright information at the top of every subsystem in design.
      mask prompts: none "No parameters"
      mask help: Place copyright information at the top of every subsystem in design.
      mask Display:
      | NxtrConf = 'Nexteer Confidential';
      | 
      | sys = bdroot; %handle for the current model ("system")
      | first = get_param(sys,'Created');
      | first = first(end-3:end);  %year is last four digits
      | 
      | last = get_param(sys,'LastModifiedDate');
      | if isempty(last)
      |     last = datestr(now,'yyyy');
      | else
      |     last = last(end-3:end);
      | end
      | 
      | if strcmp(first,last)
      |     fprintf('%s -- Copyright %s Nexteer',NxtrConf,first)
      | else
      |     fprintf('%s -- %s%s- %s Nexteer',NxtrConf,char(169),first,last)
      | end
  Terminator : Terminator
  Rx : Outport
  wires:
  Constant3/1 -> Rx/1
  Channel/1 -> Terminator/1

== system ES008A_PwrSply/PwrSply/PwrSplyPer1/SysSt = Enable/PwrSplyReadWrOrderFlg1 = 1 (Read Buffer)/No  Error - Diag Reg 0/CopyRight1 ==

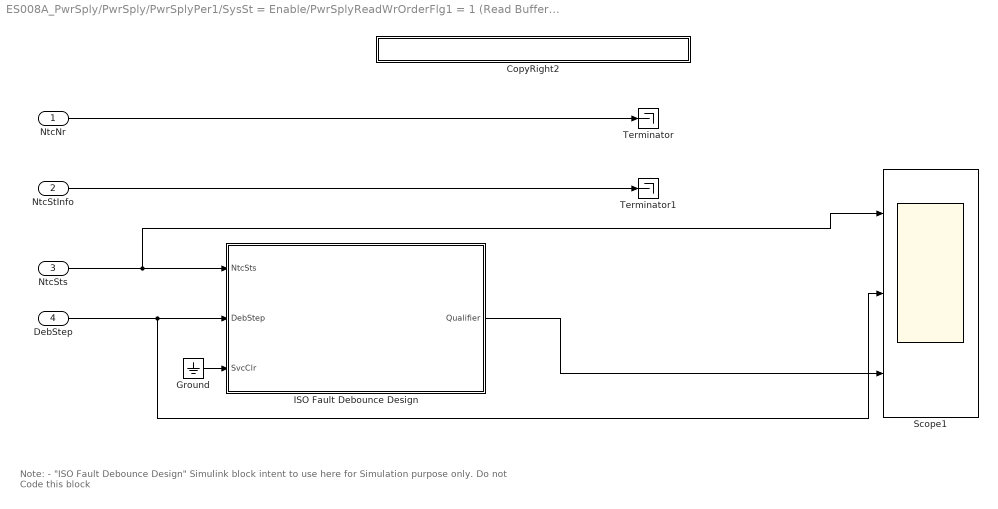
== system ES008A_PwrSply/PwrSply/PwrSplyPer1/SysSt = Enable/PwrSplyReadWrOrderFlg1 = 1 (Read Buffer)/No  Error - Diag Reg 0/SetNtcSts ==
  note: Note:
      |
      | - "ISO Fault Debounce Design" Simulink block intent to use here for Simulation purpose only. Do not Code this block
  NtcNr : Inport
  NtcStInfo : Inport  Port=2
  NtcSts : Inport  Port=3  OutDataTypeStr=uint8
  DebStep : Inport  Port=4  OutDataTypeStr=uint16
  CopyRight2 : Subsystem  Description=|  mask(Copyright Information){none=on}
      | Copyright info block.                                               
      |                                                                     
      | Place copyright information at the top of every subsystem in design.
      mask prompts: none "No parameters"
      mask help: Place copyright information at the top of every subsystem in design.
      mask Display:
      | NxtrConf = 'Nexteer Confidential';
      | 
      | sys = bdroot; %handle for the current model ("system")
      | first = get_param(sys,'Created');
      | first = first(end-3:end);  %year is last four digits
      | 
      | last = get_param(sys,'LastModifiedDate');
      | if isempty(last)
      |     last = datestr(now,'yyyy');
      | else
      |     last = last(end-3:end);
      | end
      | 
      | if strcmp(first,last)
      |     fprintf('%s -- Copyright %s Nexteer',NxtrConf,first)
      | else
      |     fprintf('%s -- %s%s- %s Nexteer',NxtrConf,char(169),first,last)
      | end
  Ground : Ground
  ISO Fault Debounce Design : Stateflow chart  TreatAsAtomicUnit=on
      settings: AttributesFormatString=|
      | Simulation Purpose Only.
      | Do Not Code this block
      | Diagnostic Manager Owns this requirement
  Scope1 : Scope  NumInputPorts=3
      settings: YMin=-5~-5~-5  YMax=5~5~5  SaveName=ScopeData5
  Terminator : Terminator
  Terminator1 : Terminator
  wires:
  Ground/1 -> ISO Fault Debounce Design/3(SvcClr)
  ISO Fault Debounce Design/1(Qualifier) -> Scope1/3
  DebStep/1 -> Scope1/2, ISO Fault Debounce Design/2(DebStep)
  NtcSts/1 -> Scope1/1, ISO Fault Debounce Design/1(NtcSts)
  NtcNr/1 -> Terminator/1
  NtcStInfo/1 -> Terminator1/1

== system ES008A_PwrSply/PwrSply/PwrSplyPer1/SysSt = Enable/PwrSplyReadWrOrderFlg1 = 1 (Read Buffer)/No  Error - Diag Reg 1/CopyRight1 ==

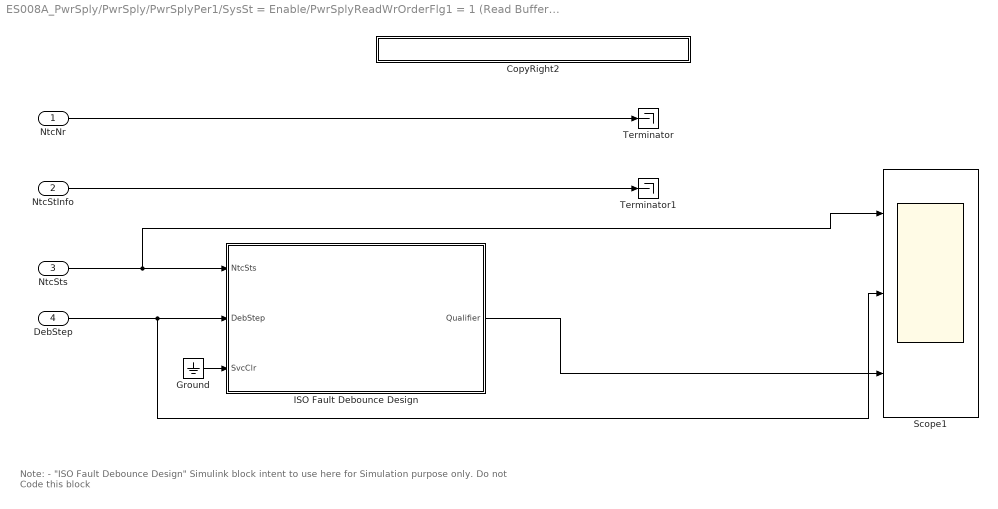
== system ES008A_PwrSply/PwrSply/PwrSplyPer1/SysSt = Enable/PwrSplyReadWrOrderFlg1 = 1 (Read Buffer)/No  Error - Diag Reg 1/SetNtcSts ==
  note: Note:
      |
      | - "ISO Fault Debounce Design" Simulink block intent to use here for Simulation purpose only. Do not Code this block
  NtcNr : Inport
  NtcStInfo : Inport  Port=2
  NtcSts : Inport  Port=3  OutDataTypeStr=uint8
  DebStep : Inport  Port=4  OutDataTypeStr=uint16
  CopyRight2 : Subsystem  Description=|  mask(Copyright Information){none=on}
      | Copyright info block.                                               
      |                                                                     
      | Place copyright information at the top of every subsystem in design.
      mask prompts: none "No parameters"
      mask help: Place copyright information at the top of every subsystem in design.
      mask Display:
      | NxtrConf = 'Nexteer Confidential';
      | 
      | sys = bdroot; %handle for the current model ("system")
      | first = get_param(sys,'Created');
      | first = first(end-3:end);  %year is last four digits
      | 
      | last = get_param(sys,'LastModifiedDate');
      | if isempty(last)
      |     last = datestr(now,'yyyy');
      | else
      |     last = last(end-3:end);
      | end
      | 
      | if strcmp(first,last)
      |     fprintf('%s -- Copyright %s Nexteer',NxtrConf,first)
      | else
      |     fprintf('%s -- %s%s- %s Nexteer',NxtrConf,char(169),first,last)
      | end
  Ground : Ground
  ISO Fault Debounce Design : Stateflow chart  TreatAsAtomicUnit=on
      settings: AttributesFormatString=|
      | Simulation Purpose Only.
      | Do Not Code this block
      | Diagnostic Manager Owns this requirement
  Scope1 : Scope  NumInputPorts=3
      settings: YMin=-5~-5~-5  YMax=5~5~5  SaveName=ScopeData5
  Terminator : Terminator
  Terminator1 : Terminator
  wires:
  NtcStInfo/1 -> Terminator1/1
  NtcNr/1 -> Terminator/1
  NtcSts/1 -> ISO Fault Debounce Design/1(NtcSts), Scope1/1
  DebStep/1 -> ISO Fault Debounce Design/2(DebStep), Scope1/2
  ISO Fault Debounce Design/1(Qualifier) -> Scope1/3
  Ground/1 -> ISO Fault Debounce Design/3(SvcClr)

== system ES008A_PwrSply/PwrSply/PwrSplyPer1/SysSt = Enable/PwrSplyReadWrOrderFlg1 = 1 (Read Buffer)/No Serial Error/CopyRight1 ==

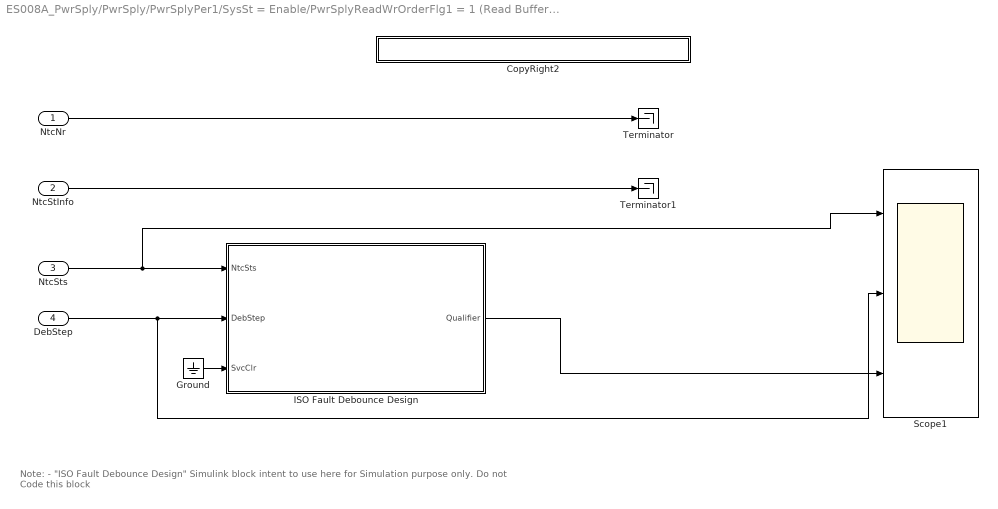
== system ES008A_PwrSply/PwrSply/PwrSplyPer1/SysSt = Enable/PwrSplyReadWrOrderFlg1 = 1 (Read Buffer)/No Serial Error/SetNtcSts ==
  note: Note:
      |
      | - "ISO Fault Debounce Design" Simulink block intent to use here for Simulation purpose only. Do not Code this block
  NtcNr : Inport
  NtcStInfo : Inport  Port=2
  NtcSts : Inport  Port=3  OutDataTypeStr=uint8
  DebStep : Inport  Port=4  OutDataTypeStr=uint16
  CopyRight2 : Subsystem  Description=|  mask(Copyright Information){none=on}
      | Copyright info block.                                               
      |                                                                     
      | Place copyright information at the top of every subsystem in design.
      mask prompts: none "No parameters"
      mask help: Place copyright information at the top of every subsystem in design.
      mask Display:
      | NxtrConf = 'Nexteer Confidential';
      | 
      | sys = bdroot; %handle for the current model ("system")
      | first = get_param(sys,'Created');
      | first = first(end-3:end);  %year is last four digits
      | 
      | last = get_param(sys,'LastModifiedDate');
      | if isempty(last)
      |     last = datestr(now,'yyyy');
      | else
      |     last = last(end-3:end);
      | end
      | 
      | if strcmp(first,last)
      |     fprintf('%s -- Copyright %s Nexteer',NxtrConf,first)
      | else
      |     fprintf('%s -- %s%s- %s Nexteer',NxtrConf,char(169),first,last)
      | end
  Ground : Ground
  ISO Fault Debounce Design : Stateflow chart  TreatAsAtomicUnit=on
      settings: AttributesFormatString=|
      | Simulation Purpose Only.
      | Do Not Code this block
      | Diagnostic Manager Owns this requirement
  Scope1 : Scope  NumInputPorts=3
      settings: YMin=-5~-5~-5  YMax=5~5~5  SaveName=ScopeData5
  Terminator : Terminator
  Terminator1 : Terminator
  wires:
  Ground/1 -> ISO Fault Debounce Design/3(SvcClr)
  ISO Fault Debounce Design/1(Qualifier) -> Scope1/3
  DebStep/1 -> Scope1/2, ISO Fault Debounce Design/2(DebStep)
  NtcSts/1 -> Scope1/1, ISO Fault Debounce Design/1(NtcSts)
  NtcNr/1 -> Terminator/1
  NtcStInfo/1 -> Terminator1/1

== system ES008A_PwrSply/PwrSply/PwrSplyPer1/SysSt = Enable/PwrSplyReadWrOrderFlg1 = 1 (Read Buffer)/Serial Error - NTCNR_0X07D/CopyRight1 ==

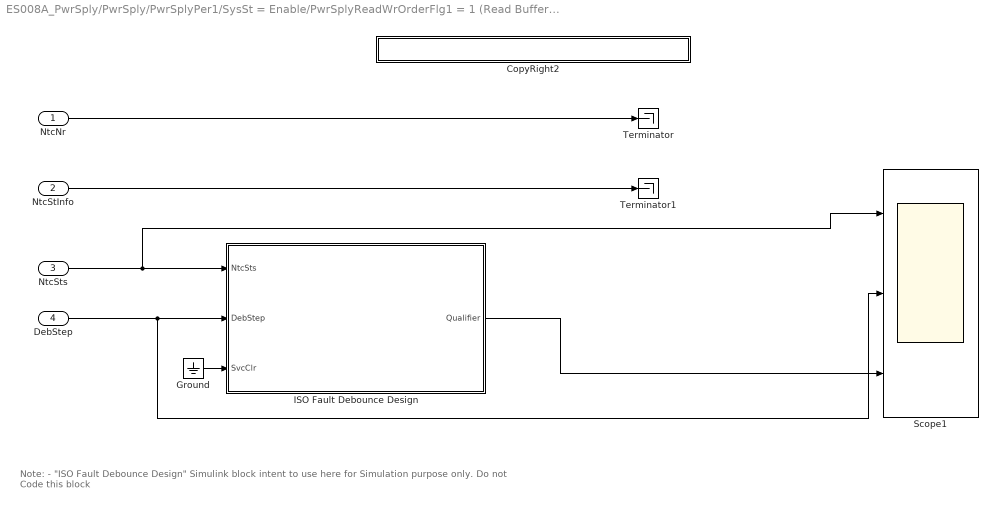
== system ES008A_PwrSply/PwrSply/PwrSplyPer1/SysSt = Enable/PwrSplyReadWrOrderFlg1 = 1 (Read Buffer)/Serial Error - NTCNR_0X07D/SetNtcSts ==
  note: Note:
      |
      | - "ISO Fault Debounce Design" Simulink block intent to use here for Simulation purpose only. Do not Code this block
  NtcNr : Inport
  NtcStInfo : Inport  Port=2
  NtcSts : Inport  Port=3  OutDataTypeStr=uint8
  DebStep : Inport  Port=4  OutDataTypeStr=uint16
  CopyRight2 : Subsystem  Description=|  mask(Copyright Information){none=on}
      | Copyright info block.                                               
      |                                                                     
      | Place copyright information at the top of every subsystem in design.
      mask prompts: none "No parameters"
      mask help: Place copyright information at the top of every subsystem in design.
      mask Display:
      | NxtrConf = 'Nexteer Confidential';
      | 
      | sys = bdroot; %handle for the current model ("system")
      | first = get_param(sys,'Created');
      | first = first(end-3:end);  %year is last four digits
      | 
      | last = get_param(sys,'LastModifiedDate');
      | if isempty(last)
      |     last = datestr(now,'yyyy');
      | else
      |     last = last(end-3:end);
      | end
      | 
      | if strcmp(first,last)
      |     fprintf('%s -- Copyright %s Nexteer',NxtrConf,first)
      | else
      |     fprintf('%s -- %s%s- %s Nexteer',NxtrConf,char(169),first,last)
      | end
  Ground : Ground
  ISO Fault Debounce Design : Stateflow chart  TreatAsAtomicUnit=on
      settings: AttributesFormatString=|
      | Simulation Purpose Only.
      | Do Not Code this block
      | Diagnostic Manager Owns this requirement
  Scope1 : Scope  NumInputPorts=3
      settings: YMin=-5~-5~-5  YMax=5~5~5  SaveName=ScopeData5
  Terminator : Terminator
  Terminator1 : Terminator
  wires:
  Ground/1 -> ISO Fault Debounce Design/3(SvcClr)
  ISO Fault Debounce Design/1(Qualifier) -> Scope1/3
  DebStep/1 -> Scope1/2, ISO Fault Debounce Design/2(DebStep)
  NtcSts/1 -> Scope1/1, ISO Fault Debounce Design/1(NtcSts)
  NtcNr/1 -> Terminator/1
  NtcStInfo/1 -> Terminator1/1

== system ES008A_PwrSply/PwrSply/PwrSplyPer1/SysSt = Enable/PwrSplyReadWrOrderFlg1 = 1 (Read Buffer)/Spi_ReadIB/CopyRight1 ==
